simulink model "ISReferenceApplication"  (R2018a)
settings: Solver=FixedStepAuto  StartTime=0  StopTime=Tend  FixedStep=0.001  RelTol=5e-3
model workspace (MAT data in the model file):
  A_mu = 10
  B_reff = 8.386
  Cz = 7766.25
  DCT_Param : struct (value not decoded)
  D_reff = 0.25826
  Downshift_Speeds = [9.5625 12.9375 16.3125 19.6875 23.0625 26.4375 29.8125 33.1875 36.5625 39.9375 43.3125 46.6875 ... (28 elements, 4x7)]
  Pedal_Positions = [0.1 0.4 0.5 0.9]
  SUS : struct (value not decoded)
  Upshift_Speeds = [12.9375 16.3125 19.6875 33 26.4375 29.8125 33.1875 52.5 39.9375 43.3125 46.6875 77.25 ... (28 elements, 4x7)]
  VEH : struct (value not decoded)
  V_o = 16.7
  V_xlow = 1
  WH : struct (value not decoded)
  a = 1.4
  alpha_max = 1.5
  alpha_min = -1.5
  b = 1.8
  c_zo = 209651
  epsilon = 0.1
  h = 0.134
  path : struct (value not decoded)
  pio = 220000
  q_Fcx = 0
  q_Fz2 = 15.4
  q_Fzy = 0
  q_reo = 0.9974
  q_sx1 = -0.007764
  q_sx10 = 0.2824
  q_sx11 = 5.349
  q_sx12 = 0
  q_sx13 = 0
  q_sx14 = 0
  q_sx2 = 1.1915
  q_sx3 = 0.013948
  q_sx4 = 4.912
  q_sx5 = 1.02
  q_sx6 = 22.83
  q_sx7 = 0.7104
  q_sx8 = -0.023393
  q_sx9 = 0.6581
  q_sy1 = 0.00702
  q_sy2 = 0
  q_sy3 = 0.001515
  q_sy4 = 8.514e-05
  q_sy5 = 0
  q_sy6 = 0
  q_sy7 = 0.9008
  q_sy8 = -0.4089
  q_v1 = 0.0007742
  q_v2 = 0.04667
  r_Bx1 = 12.531
  r_Bx2 = 9.532
  r_Bx3 = 0
  r_By1 = 10.615
  r_By2 = 7.705
  r_By3 = 3.433e-06
  r_By4 = 0
  r_Cx1 = 1.019
  r_Cy1 = 1.0585
  r_Ex1 = -0.4487
  r_Ex2 = -0.4726
  r_Ey1 = 0.3132
  r_Ey2 = 7.63e-06
  r_Hx1 = 0.0002374
  r_Hy1 = 0.011646
  r_Hy2 = 7.63e-06
  r_Vy1 = 0.05654
  r_Vy2 = 7.63e-06
  r_Vy3 = 0
  r_Vy4 = 99.9
  r_Vy5 = 2
  r_Vy6 = 15.814
  r_o = 0.3135
  vehWidth = 2
  w = 1
undefined symbols (not defined in the file): Cok_1, Cok_2, Cok_3, Cok_4, Cok_5, Cok_6, Cok_7, Cok_8, Cok_9, Cout_1, Cout_2, Cout_3, Cout_4, Cout_5, Cout_6, Cout_7, Cout_8, Cout_9, Dout_1, Dout_2, Dout_3, Dout_4, Dout_5, Dout_6, Dout_7, Dout_8, Dout_9, F_1, F_2, F_3, F_4, F_5, F_6, F_7, F_8, F_9, Gd_1, Gd_2, Gd_3, Gd_4, Gd_5, Gd_6, Gd_7, Gd_8, Gd_9, Gok_1, Gok_2, Gok_3, Gok_4, Gok_5, Gok_6, Gok_7, Gok_8, Gok_9, Hd_1, Hd_2, Hd_3, Hd_4, Hd_5, Hd_6 ... (+64)
(part 3 of 3)

== system ISReferenceApplication/Subsystem_7/Subsystem/VH2P ==
  Velocities : Inport
  HeadingAngles : Inport  Port=2
  Iintial Velocities : Inport  Port=3
  Iintial HeadingAngles : Inport  Port=4
  Initial position : Inport  Port=5
  select_overlap : Inport  Port=6
  Delay1 : Delay  DelayLength=1  InitialConditionSource=Input port  InitialCondition=0  ExternalReset=Rising  SampleTime=Ts
      settings: InputPortMap=u0,r5,p4
  Delay2 : Delay  DelayLength=1  InitialConditionSource=Input port  InitialCondition=0  ExternalReset=Rising  SampleTime=Ts
      settings: InputPortMap=u0,r5,p4
  Delay3 : Delay  DelayLength=1  InitialConditionSource=Input port  InitialCondition=0  ExternalReset=Rising  SampleTime=Ts
      settings: InputPortMap=u0,r5,p4
  From Workspace : FromWorkspace  VariableName=T_sim  SampleTime=Ts
  Unit Delay3 : UnitDelay  SampleTime=Ts
  YV2P : MATLAB Function  TreatAsAtomicUnit=on  SystemSampleTime=Ts
  Position : Outport
  wires:
  Velocities/1 -> YV2P/1(Velocity), Delay1/1
  HeadingAngles/1 -> Delay3/1, YV2P/3(Yaw)
  Delay2/1 -> YV2P/7(Lastpostion)
  Initial position/1 -> Delay2/3
  Iintial Velocities/1 -> Delay1/3
  Iintial HeadingAngles/1 -> Delay3/3
  From Workspace/1 -> YV2P/5(Tsim), Unit Delay3/1
  Delay1/1 -> YV2P/2(LastVelocity)
  Delay3/1 -> YV2P/4(LastYaw)
  Unit Delay3/1 -> YV2P/6(LastTsim)
  YV2P/1(Position) -> Delay2/1, Position/1
  select_overlap/1 -> Delay2/2, Delay1/2, Delay3/2

== system ISReferenceApplication/Subsystem_7/Subsystem/YV_update ==
  XY_sim : Inport
  Velocity_sim : Inport  Port=2
  Heading_sim : Inport  Port=3
  Constant : Constant  Value=Ts  SampleTime=Ts
  From Workspace1 : FromWorkspace  VariableName=T_sim  SampleTime=Ts
  From Workspace3 : FromWorkspace  VariableName=XY_Ref_Upd  SampleTime=Ts
  YV_update : MATLAB Function  TreatAsAtomicUnit=on  SystemSampleTime=Ts
  Velocity_updated : Outport
  Heading_updated : Outport  Port=2
  wires:
  YV_update/1(Velocity_updated) -> Velocity_updated/1
  From Workspace3/1 -> YV_update/1(XYplot_ref)
  YV_update/2(Heading_updated) -> Heading_updated/1
  From Workspace1/1 -> YV_update/6(Tsim)
  XY_sim/1 -> YV_update/2(XYplot_sim)
  Velocity_sim/1 -> YV_update/3(Velocity_sim)
  Heading_sim/1 -> YV_update/4(Heading_sim)
  Constant/1 -> YV_update/5(Ts)

== system ISReferenceApplication/Subsystem_8/Subsystem/MPC_of_simulator_8 ==
  Velocity_updated : Inport  SampleTime=Ts  LockScale=on
  Heading_updated : Inport  Port=2  SampleTime=Ts  LockScale=on
  select_MPC : Inport  Port=3  SampleTime=Ts  LockScale=on
  select_overlap : Inport  Port=4  SampleTime=Ts  LockScale=on
  U(k-1) : Inport  Port=5  SampleTime=Ts  LockScale=on
  Xhat : Inport  Port=6
  Clock : Clock
  Constant1 : Constant  Value=M  VectorParams1D=off  SampleTime=-1
  Constant2 : Constant  Value=Np  SampleTime=-1
  Constant3 : Constant  Value=JE_8  VectorParams1D=off  SampleTime=-1
  Constant4 : Constant  Value=Qc_8  VectorParams1D=off  SampleTime=-1
  Constant5 : Constant  Value=phi_8  VectorParams1D=off  SampleTime=-1
  Constant6 : Constant  Value=Tend  SampleTime=-1
  F_Middle : Gain  Gain=F_8  Multiplication=Matrix(K*u) (u vector)
  From Workspace6 : FromWorkspace  VariableName=Rs  SampleTime=Ts
  HQP : MATLAB Function  TreatAsAtomicUnit=on  SystemSampleTime=Ts
  Resettable Delay2 : Delay  DelayLength=1  InitialConditionSource=Input port  ExternalReset=Rising  SampleTime=Ts
      settings: InputPortMap=u0,r5,p4
  r(k+1) : Outport
  U : Outport  Port=2
  wires:
  HQP/2(U) -> Resettable Delay2/1, U/1
  Xhat/1 -> F_Middle/1
  Constant4/1 -> HQP/4(Qc)
  Constant5/1 -> HQP/2(phi)
  Constant3/1 -> HQP/1(JE)
  Constant2/1 -> HQP/6(Np)
  Constant1/1 -> HQP/5(M)
  Clock/1 -> HQP/10(Tsim)
  F_Middle/1 -> HQP/3(Fxh)
  From Workspace6/1 -> HQP/9(Rs)
  Heading_updated/1 -> HQP/7(Heading_updated)
  Velocity_updated/1 -> HQP/8(Velocity_updated)
  HQP/1(r) -> r(k+1)/1
  select_MPC/1 -> HQP/11(select_MPC)
  Resettable Delay2/1 -> HQP/13(U_delay)
  select_overlap/1 -> Resettable Delay2/2
  U(k-1)/1 -> Resettable Delay2/3
  Constant6/1 -> HQP/12(Tend)

== system ISReferenceApplication/Subsystem_8/Subsystem/VH2P ==
  Velocities : Inport
  HeadingAngles : Inport  Port=2
  Iintial Velocities : Inport  Port=3
  Iintial HeadingAngles : Inport  Port=4
  Initial position : Inport  Port=5
  select_overlap : Inport  Port=6
  Delay1 : Delay  DelayLength=1  InitialConditionSource=Input port  InitialCondition=0  ExternalReset=Rising  SampleTime=Ts
      settings: InputPortMap=u0,r5,p4
  Delay2 : Delay  DelayLength=1  InitialConditionSource=Input port  InitialCondition=0  ExternalReset=Rising  SampleTime=Ts
      settings: InputPortMap=u0,r5,p4
  Delay3 : Delay  DelayLength=1  InitialConditionSource=Input port  InitialCondition=0  ExternalReset=Rising  SampleTime=Ts
      settings: InputPortMap=u0,r5,p4
  From Workspace : FromWorkspace  VariableName=T_sim  SampleTime=Ts
  Unit Delay3 : UnitDelay  SampleTime=Ts
  YV2P : MATLAB Function  TreatAsAtomicUnit=on  SystemSampleTime=Ts
  Position : Outport
  wires:
  Velocities/1 -> YV2P/1(Velocity), Delay1/1
  HeadingAngles/1 -> Delay3/1, YV2P/3(Yaw)
  Delay2/1 -> YV2P/7(Lastpostion)
  Initial position/1 -> Delay2/3
  Iintial Velocities/1 -> Delay1/3
  Iintial HeadingAngles/1 -> Delay3/3
  From Workspace/1 -> YV2P/5(Tsim), Unit Delay3/1
  Delay1/1 -> YV2P/2(LastVelocity)
  Delay3/1 -> YV2P/4(LastYaw)
  Unit Delay3/1 -> YV2P/6(LastTsim)
  YV2P/1(Position) -> Delay2/1, Position/1
  select_overlap/1 -> Delay2/2, Delay1/2, Delay3/2

== system ISReferenceApplication/Subsystem_8/Subsystem/YV_update ==
  XY_sim : Inport
  Velocity_sim : Inport  Port=2
  Heading_sim : Inport  Port=3
  Constant : Constant  Value=Ts  SampleTime=Ts
  From Workspace1 : FromWorkspace  VariableName=T_sim  SampleTime=Ts
  From Workspace3 : FromWorkspace  VariableName=XY_Ref_Upd  SampleTime=Ts
  YV_update : MATLAB Function  TreatAsAtomicUnit=on  SystemSampleTime=Ts
  Velocity_updated : Outport
  Heading_updated : Outport  Port=2
  wires:
  YV_update/1(Velocity_updated) -> Velocity_updated/1
  From Workspace3/1 -> YV_update/1(XYplot_ref)
  YV_update/2(Heading_updated) -> Heading_updated/1
  From Workspace1/1 -> YV_update/6(Tsim)
  XY_sim/1 -> YV_update/2(XYplot_sim)
  Velocity_sim/1 -> YV_update/3(Velocity_sim)
  Heading_sim/1 -> YV_update/4(Heading_sim)
  Constant/1 -> YV_update/5(Ts)

== system ISReferenceApplication/Subsystem_9/Subsystem/MPC_of_simulator_9 ==
  Velocity_updated : Inport  SampleTime=Ts  LockScale=on
  Heading_updated : Inport  Port=2  SampleTime=Ts  LockScale=on
  select_MPC : Inport  Port=3  SampleTime=Ts  LockScale=on
  select_overlap : Inport  Port=4  SampleTime=Ts  LockScale=on
  U(k-1) : Inport  Port=5  SampleTime=Ts  LockScale=on
  Xhat : Inport  Port=6
  Clock : Clock
  Constant1 : Constant  Value=M  VectorParams1D=off  SampleTime=-1
  Constant2 : Constant  Value=Np  SampleTime=-1
  Constant3 : Constant  Value=JE_9  VectorParams1D=off  SampleTime=-1
  Constant4 : Constant  Value=Qc_9  VectorParams1D=off  SampleTime=-1
  Constant5 : Constant  Value=phi_9  VectorParams1D=off  SampleTime=-1
  Constant6 : Constant  Value=Tend  SampleTime=-1
  F_Middle : Gain  Gain=F_9  Multiplication=Matrix(K*u) (u vector)
  From Workspace6 : FromWorkspace  VariableName=Rs  SampleTime=Ts
  HQP : MATLAB Function  TreatAsAtomicUnit=on  SystemSampleTime=Ts
  Resettable Delay2 : Delay  DelayLength=1  InitialConditionSource=Input port  ExternalReset=Rising  SampleTime=Ts
      settings: InputPortMap=u0,r5,p4
  r(k+1) : Outport
  U : Outport  Port=2
  wires:
  HQP/2(U) -> Resettable Delay2/1, U/1
  Xhat/1 -> F_Middle/1
  Constant4/1 -> HQP/4(Qc)
  Constant5/1 -> HQP/2(phi)
  Constant3/1 -> HQP/1(JE)
  Constant2/1 -> HQP/6(Np)
  Constant1/1 -> HQP/5(M)
  Clock/1 -> HQP/10(Tsim)
  F_Middle/1 -> HQP/3(Fxh)
  From Workspace6/1 -> HQP/9(Rs)
  Heading_updated/1 -> HQP/7(Heading_updated)
  Velocity_updated/1 -> HQP/8(Velocity_updated)
  HQP/1(r) -> r(k+1)/1
  select_MPC/1 -> HQP/11(select_MPC)
  Resettable Delay2/1 -> HQP/13(U_delay)
  select_overlap/1 -> Resettable Delay2/2
  U(k-1)/1 -> Resettable Delay2/3
  Constant6/1 -> HQP/12(Tend)

== system ISReferenceApplication/Subsystem_9/Subsystem/VH2P ==
  Velocities : Inport
  HeadingAngles : Inport  Port=2
  Iintial Velocities : Inport  Port=3
  Iintial HeadingAngles : Inport  Port=4
  Initial position : Inport  Port=5
  select_overlap : Inport  Port=6
  Delay1 : Delay  DelayLength=1  InitialConditionSource=Input port  InitialCondition=0  ExternalReset=Rising  SampleTime=Ts
      settings: InputPortMap=u0,r5,p4
  Delay2 : Delay  DelayLength=1  InitialConditionSource=Input port  InitialCondition=0  ExternalReset=Rising  SampleTime=Ts
      settings: InputPortMap=u0,r5,p4
  Delay3 : Delay  DelayLength=1  InitialConditionSource=Input port  InitialCondition=0  ExternalReset=Rising  SampleTime=Ts
      settings: InputPortMap=u0,r5,p4
  From Workspace : FromWorkspace  VariableName=T_sim  SampleTime=Ts
  Unit Delay3 : UnitDelay  SampleTime=Ts
  YV2P : MATLAB Function  TreatAsAtomicUnit=on  SystemSampleTime=Ts
  Position : Outport
  wires:
  Velocities/1 -> YV2P/1(Velocity), Delay1/1
  HeadingAngles/1 -> Delay3/1, YV2P/3(Yaw)
  Delay2/1 -> YV2P/7(Lastpostion)
  Initial position/1 -> Delay2/3
  Iintial Velocities/1 -> Delay1/3
  Iintial HeadingAngles/1 -> Delay3/3
  From Workspace/1 -> YV2P/5(Tsim), Unit Delay3/1
  Delay1/1 -> YV2P/2(LastVelocity)
  Delay3/1 -> YV2P/4(LastYaw)
  Unit Delay3/1 -> YV2P/6(LastTsim)
  YV2P/1(Position) -> Delay2/1, Position/1
  select_overlap/1 -> Delay2/2, Delay1/2, Delay3/2

== system ISReferenceApplication/Subsystem_9/Subsystem/YV_update ==
  XY_sim : Inport
  Velocity_sim : Inport  Port=2
  Heading_sim : Inport  Port=3
  Constant : Constant  Value=Ts  SampleTime=Ts
  From Workspace1 : FromWorkspace  VariableName=T_sim  SampleTime=Ts
  From Workspace3 : FromWorkspace  VariableName=XY_Ref_Upd  SampleTime=Ts
  YV_update : MATLAB Function  TreatAsAtomicUnit=on  SystemSampleTime=Ts
  Velocity_updated : Outport
  Heading_updated : Outport  Port=2
  wires:
  YV_update/1(Velocity_updated) -> Velocity_updated/1
  From Workspace3/1 -> YV_update/1(XYplot_ref)
  YV_update/2(Heading_updated) -> Heading_updated/1
  From Workspace1/1 -> YV_update/6(Tsim)
  XY_sim/1 -> YV_update/2(XYplot_sim)
  Velocity_sim/1 -> YV_update/3(Velocity_sim)
  Heading_sim/1 -> YV_update/4(Heading_sim)
  Constant/1 -> YV_update/5(Ts)

== matlab function ISReferenceApplication/Subsystem_6/Subsystem/MPC_of_simulator_6/HQP ==
  data: r output; JE input; phi input; Fxh input; Qc input; U output; M input; Np input; Heading_updated input; Velocity_updated input; Rs input; Tsim input; select_MPC input; Tend input; U_delay input; select_overlap input
function [r,U] = HQP(JE ,phi,Fxh ,Qc ,M ,Np,Heading_updated ,Velocity_updated ,Rs ,Tsim, select_MPC, Tend, U_delay, select_overlap)
u1_max = 3*pi; u1_min = -3*pi;
u2_max =  1; u2_min = -1;
du1_inc = 3*pi;du1_dec = 3*pi;
du2_inc =  1;du2_dec =  1;
U_max = []; U_min = [];
for i = 1:Np
    U_max = [U_max; [u1_max; u2_max]];
    U_min = [U_min; [-u1_min; -u2_min]];
end

dU_plus = []; dU_minus = [];
for i = 1:Np
    dU_plus = [dU_plus; [U_delay(1) + du1_inc; U_delay(2) + du2_inc]];
    dU_minus = [dU_minus; [-U_delay(1) + du1_dec; -U_delay(2) + du2_dec;]];
end
N = [U_max;
      U_min;
      dU_plus;
      dU_minus;          
     ];
if Tsim > 0 %&& select_MPC~=1 %&& select_overlap~=1 
    for i = 1: Np
        Rs(2*i,:) = Heading_updated(i,:);
        Rs(2*i-1,:) = Velocity_updated(i,:);
    end
end
JF = -2*phi'*Qc*(Rs-Fxh);
[u,lambda]= HQP(JE,JF,M,N);
U = u(1:2);
r = Rs(1:2,:);
end

== matlab function ISReferenceApplication/Subsystem_6/Subsystem/VH2P/YV2P ==
  data: Velocity input; LastVelocity input; Yaw input; LastYaw input; Tsim input; LastTsim input; Lastpostion input; Position output
function Position  = YV2P(Velocity, LastVelocity, Yaw, LastYaw, Tsim, LastTsim, Lastpostion)
if Tsim >= 0.1
    Position = zeros(2,1);
    X0 = Lastpostion(1,:); Y0 = Lastpostion(2,:);
    Vx = [LastVelocity*cos(LastYaw); Velocity*cos(Yaw)];
    Vy = [LastVelocity*sin(LastYaw); Velocity*sin(Yaw)];
    Yaw_sim = [LastYaw; Yaw];
    T_sample =[LastTsim; Tsim];
    [ X_tmp, Y_tmp] = YV2P( T_sample, X0, Y0, Vx, Vy, Yaw_sim, zeros(2,1) );
    Position = [X_tmp(end,:); Y_tmp(end,:)];
else
    Position = [0; 0];
end

end

== matlab function ISReferenceApplication/Subsystem_6/Subsystem/YV_update/YV_update ==
  data: XYplot_ref input; Velocity_updated output; XYplot_sim input; Velocity_sim input; Heading_sim input; Ts input; Tsim input; Heading_updated output
function [Velocity_updated, Heading_updated] = VY_update(XYplot_ref, XYplot_sim, Velocity_sim, Heading_sim, Ts, Tsim)
Np = 6;
 disp(sprintf('Simulation time : %2.1f sec',Tsim)) 
 Heading_updated = zeros(Np,1); Velocity_updated = zeros(Np,1);
coder.extrinsic('P2YV');
T = []; 
for j = 1:Np+1
    T = [T; Tsim+(j-1)*Ts];
end
X = [];
for i = 1:Np
    X = [X; XYplot_ref(2*i-1,:)];
end
Y = [];
for i = 1:Np
    Y = [Y; XYplot_ref(2*i,:)];
end

X = [XYplot_sim(1,:); X];
Y = [XYplot_sim(2,:); Y];   
Vx0 = Velocity_sim*cos(Heading_sim);
Vy0 = Velocity_sim*sin(Heading_sim);
Yaw0 = Heading_sim;

[Velocity_updated, Heading_updated] = P2YV(0,0, T , X , Y , Vx0 , Vy0 , Yaw0, Np, 0, 0 );
end

== matlab function ISReferenceApplication/Subsystem_3/Subsystem/MPC_of_simulator_3/HQP ==
  data: r output; JE input; phi input; Fxh input; Qc input; U output; M input; Np input; Heading_updated input; Velocity_updated input; Rs input; Tsim input; select_MPC input; Tend input; U_delay input; select_overlap input
function [r,U] = HQP(JE ,phi,Fxh ,Qc ,M ,Np,Heading_updated ,Velocity_updated ,Rs ,Tsim, select_MPC, Tend, U_delay, select_overlap)
u1_max = 3*pi; u1_min = -3*pi;
u2_max =  1; u2_min = -1;
du1_inc = 3*pi;du1_dec = 3*pi;
du2_inc =  1;du2_dec =  1;
U_max = []; U_min = [];
for i = 1:Np
    U_max = [U_max; [u1_max; u2_max]];
    U_min = [U_min; [-u1_min; -u2_min]];
end

dU_plus = []; dU_minus = [];
for i = 1:Np
    dU_plus = [dU_plus; [U_delay(1) + du1_inc; U_delay(2) + du2_inc]];
    dU_minus = [dU_minus; [-U_delay(1) + du1_dec; -U_delay(2) + du2_dec;]];
end
N = [U_max;
      U_min;
      dU_plus;
      dU_minus;          
     ];
if Tsim > 0 %&& select_overlap~=1 && select_MPC~=1
    for i = 1: Np
        Rs(2*i,:) = Heading_updated(i,:);
        Rs(2*i-1,:) = Velocity_updated(i,:);
    end
end
JF = -2*phi'*Qc*(Rs-Fxh);
[u,lambda]= HQP(JE,JF,M,N);

U = u(1:2);
r = Rs(1:2,:);
end

== matlab function ISReferenceApplication/Subsystem_3/Subsystem/VH2P/YV2P ==
  data: Velocity input; LastVelocity input; Yaw input; LastYaw input; Tsim input; LastTsim input; Lastpostion input; Position output
function Position  = YV2P(Velocity, LastVelocity, Yaw, LastYaw, Tsim, LastTsim, Lastpostion)
if Tsim >= 0.1
    Position = zeros(2,1);
    X0 = Lastpostion(1,:); Y0 = Lastpostion(2,:);
    Vx = [LastVelocity*cos(LastYaw); Velocity*cos(Yaw)];
    Vy = [LastVelocity*sin(LastYaw); Velocity*sin(Yaw)];
    Yaw_sim = [LastYaw; Yaw];
    T_sample =[LastTsim; Tsim];
    [ X_tmp, Y_tmp] = YV2P( T_sample, X0, Y0, Vx, Vy, Yaw_sim, zeros(2,1) );
    Position = [X_tmp(end,:); Y_tmp(end,:)];
else
    Position = [0; 0];
end

end

== matlab function ISReferenceApplication/Subsystem_4/Subsystem/MPC_of_simulator_4/HQP ==
  data: r output; JE input; phi input; Fxh input; Qc input; U output; M input; Np input; Heading_updated input; Velocity_updated input; Rs input; Tsim input; select_MPC input; Tend input; U_delay input; select_overlap input
function [r,U] = HQP(JE ,phi,Fxh ,Qc ,M ,Np,Heading_updated ,Velocity_updated ,Rs ,Tsim, select_MPC, Tend, U_delay, select_overlap)
u1_max = 3*pi; u1_min = -3*pi;
u2_max =  1; u2_min = -1;
du1_inc = 3*pi;du1_dec = 3*pi;
du2_inc =  1;du2_dec =  1;
U_max = []; U_min = [];
for i = 1:Np
    U_max = [U_max; [u1_max; u2_max]];
    U_min = [U_min; [-u1_min; -u2_min]];
end

dU_plus = []; dU_minus = [];
for i = 1:Np
    dU_plus = [dU_plus; [U_delay(1) + du1_inc; U_delay(2) + du2_inc]];
    dU_minus = [dU_minus; [-U_delay(1) + du1_dec; -U_delay(2) + du2_dec;]];
end
N = [U_max;
      U_min;
      dU_plus;
      dU_minus;          
     ];
 
if Tsim > 0 && select_MPC~=1 %&& select_overlap~=1
    for i = 1: Np
        Rs(2*i,:) = Heading_updated(i,:);
        Rs(2*i-1,:) = Velocity_updated(i,:);
    end
end

JF = -2*phi'*Qc*(Rs-Fxh);
[u,lambda]= HQP(JE,JF,M,N);
U = u(1:2);
r = Rs(1:2,:);
end

== matlab function ISReferenceApplication/Subsystem_5/Subsystem/MPC_of_simulator_5/HQP ==
  data: r output; JE input; phi input; Fxh input; Qc input; U output; M input; Np input; Heading_updated input; Velocity_updated input; Rs input; Tsim input; select_MPC input; Tend input; U_delay input; select_overlap input
function [r,U] = HQP(JE ,phi,Fxh ,Qc ,M ,Np,Heading_updated ,Velocity_updated ,Rs ,Tsim, select_MPC, Tend, U_delay, select_overlap)
u1_max = 3*pi; u1_min = -3*pi;
u2_max =  1; u2_min = -1;
du1_inc = 3*pi;du1_dec = 3*pi;
du2_inc =  1;du2_dec =  1;
U_max = []; U_min = [];
for i = 1:Np
    U_max = [U_max; [u1_max; u2_max]];
    U_min = [U_min; [-u1_min; -u2_min]];
end

dU_plus = []; dU_minus = [];
for i = 1:Np
    dU_plus = [dU_plus; [U_delay(1) + du1_inc; U_delay(2) + du2_inc]];
    dU_minus = [dU_minus; [-U_delay(1) + du1_dec; -U_delay(2) + du2_dec;]];
end
N = [U_max;
      U_min;
      dU_plus;
      dU_minus;          
     ];
if Tsim > 0 %&& select_overlap~=1 && select_MPC~=1
    for i = 1: Np
        Rs(2*i,:) = Heading_updated(i,:);
        Rs(2*i-1,:) = Velocity_updated(i,:);
    end
end
JF = -2*phi'*Qc*(Rs-Fxh);
[u,lambda]= HQP(JE,JF,M,N);
U = u(1:2);
r = Rs(1:2,:);
end

== matlab function ISReferenceApplication/Subsystem_7/Subsystem/MPC_of_simulator_7/HQP ==
  data: r output; JE input; phi input; Fxh input; Qc input; U output; M input; Np input; Heading_updated input; Velocity_updated input; Rs input; Tsim input; select_MPC input; Tend input; U_delay input; select_overlap input
function [r,U] = HQP(JE ,phi,Fxh ,Qc ,M ,Np,Heading_updated ,Velocity_updated ,Rs ,Tsim, select_MPC, Tend, U_delay, select_overlap)
u1_max = 3*pi; u1_min = -3*pi;
u2_max =  1; u2_min = -1;
du1_inc = 3*pi;du1_dec = 3*pi;
du2_inc =  1;du2_dec =  1;
U_max = []; U_min = [];
for i = 1:Np
    U_max = [U_max; [u1_max; u2_max]];
    U_min = [U_min; [-u1_min; -u2_min]];
end

dU_plus = []; dU_minus = [];
for i = 1:Np
    dU_plus = [dU_plus; [U_delay(1) + du1_inc; U_delay(2) + du2_inc]];
    dU_minus = [dU_minus; [-U_delay(1) + du1_dec; -U_delay(2) + du2_dec;]];
end
N = [U_max;
      U_min;
      dU_plus;
      dU_minus;          
     ];
if Tsim > 0 %&& select_overlap~=1 && select_MPC~=1
    for i = 1: Np
        Rs(2*i,:) = Heading_updated(i,:);
        Rs(2*i-1,:) = Velocity_updated(i,:);
    end
end
JF = -2*phi'*Qc*(Rs-Fxh);
[u,lambda]= HQP(JE,JF,M,N);
U = u(1:2);
r = Rs(1:2,:);
end

== matlab function ISReferenceApplication/Subsystem_8/Subsystem/MPC_of_simulator_8/HQP ==
  data: r output; JE input; phi input; Fxh input; Qc input; U output; M input; Np input; Heading_updated input; Velocity_updated input; Rs input; Tsim input; select_MPC input; Tend input; U_delay input; select_overlap input
function [r,U] = HQP(JE ,phi,Fxh ,Qc ,M ,Np,Heading_updated ,Velocity_updated ,Rs ,Tsim, select_MPC, Tend, U_delay, select_overlap)
u1_max = 3*pi; u1_min = -3*pi;
u2_max =  1; u2_min = -1;
du1_inc = 3*pi;du1_dec = 3*pi;
du2_inc =  1;du2_dec =  1;
U_max = []; U_min = [];
for i = 1:Np
    U_max = [U_max; [u1_max; u2_max]];
    U_min = [U_min; [-u1_min; -u2_min]];
end

dU_plus = []; dU_minus = [];
for i = 1:Np
    dU_plus = [dU_plus; [U_delay(1) + du1_inc; U_delay(2) + du2_inc]];
    dU_minus = [dU_minus; [-U_delay(1) + du1_dec; -U_delay(2) + du2_dec;]];
end
N = [U_max;
      U_min;
      dU_plus;
      dU_minus;          
     ];
if Tsim > 0 %&& select_overlap~=1 && select_MPC~=1
    for i = 1: Np
        Rs(2*i,:) = Heading_updated(i,:);
        Rs(2*i-1,:) = Velocity_updated(i,:);
    end
end
JF = -2*phi'*Qc*(Rs-Fxh);
[u,lambda]= HQP(JE,JF,M,N);
U = u(1:2);
r = Rs(1:2,:);
end

== matlab function ISReferenceApplication/Subsystem_9/Subsystem/MPC_of_simulator_9/HQP ==
  data: r output; JE input; phi input; Fxh input; Qc input; U output; M input; Np input; Heading_updated input; Velocity_updated input; Rs input; Tsim input; select_MPC input; Tend input; U_delay input
function [r,U] = HQP(JE ,phi,Fxh ,Qc ,M ,Np,Heading_updated ,Velocity_updated ,Rs ,Tsim, select_MPC, Tend, U_delay)
u1_max = 3*pi; u1_min = -3*pi;
u2_max =  1; u2_min = -1;
du1_inc = 3*pi;du1_dec = 3*pi;
du2_inc =  1;du2_dec =  1;
U_max = []; U_min = [];
for i = 1:Np
    U_max = [U_max; [u1_max; u2_max]];
    U_min = [U_min; [-u1_min; -u2_min]];
end

dU_plus = []; dU_minus = [];
for i = 1:Np
    dU_plus = [dU_plus; [U_delay(1) + du1_inc; U_delay(2) + du2_inc]];
    dU_minus = [dU_minus; [-U_delay(1) + du1_dec; -U_delay(2) + du2_dec;]];
end
N = [U_max;
      U_min;
      dU_plus;
      dU_minus;          
     ];
if Tsim > 0
    for i = 1: Np
        Rs(2*i,:) = Heading_updated(i,:);
        Rs(2*i-1,:) = Velocity_updated(i,:);
    end
end
JF = -2*phi'*Qc*(Rs-Fxh);
[u,lambda]= HQP(JE,JF,M,N);
U = u(1:2);
r = Rs(1:2,:);
end

== matlab function ISReferenceApplication/Mpc_block1/Mpc ==
  data: U_delay input; select_MPC input; JE input; JF_part input; Fxh input; M input; Np input; U_min input; U_max input; Heading_updated input; Velocity_updated input; Rs input; Tsim input; U output; r output; lambda output; Tend input; Ts input
function [U, r, lambda] = ABC(U_delay, select_MPC, JE, JF_part, Fxh, M, Np, U_min, U_max, Heading_updated, Velocity_updated, Rs, Tsim, Tend, Ts)
U = zeros(2,1);
du1_inc = 3*pi;du1_dec = 3*pi;
du2_inc = 1;du2_dec = 1;
dU_plus = []; dU_minus = [];
for i = 1:Np
    dU_plus = [dU_plus; [U_delay(1) + du1_inc; U_delay(2) + du2_inc]];
    dU_minus = [dU_minus; [-U_delay(1) + du1_dec; -U_delay(2) + du2_dec;]];
end

N = [U_max;
      U_min;
      dU_plus;
      dU_minus;          
     ];
 
if Tsim > 0 && select_MPC ~= 4 %&& select_MPC ~= 5 %&& select_MPC ~= 6 %&& select_MPC~=8
    for i = 1: Np  
        Rs(2*i-1,:) = Velocity_updated(i,:);
        Rs(2*i,:) = Heading_updated(i,:);
    end
end

JF = JF_part*(Rs-Fxh);
[u,lambda]= HQP(JE,JF,M,N);
U = u(1:2);
r = Rs(1:2,:);
end

== matlab function ISReferenceApplication/Subsystem_1/Subsystem/MPC_of_simulator_1/HQP ==
  data: r output; JE input; phi input; Fxh input; Qc input; U output; M input; Np input; Heading_updated input; Velocity_updated input; Rs input; Tsim input; select_MPC input; Tend input; U_delay input; select_overlap input
function [r,U] = HQP(JE ,phi,Fxh ,Qc ,M ,Np,Heading_updated ,Velocity_updated ,Rs ,Tsim, select_MPC, Tend, U_delay, select_overlap)
u1_max = 3*pi; u1_min = -3*pi;
u2_max =  1; u2_min = -1;
du1_inc = 3*pi;du1_dec = 3*pi;
du2_inc =  1;du2_dec =  1;
U_max = []; U_min = [];
for i = 1:Np
    U_max = [U_max; [u1_max; u2_max]];
    U_min = [U_min; [-u1_min; -u2_min]];
end

dU_plus = []; dU_minus = [];
for i = 1:Np
    dU_plus = [dU_plus; [U_delay(1) + du1_inc; U_delay(2) + du2_inc]];
    dU_minus = [dU_minus; [-U_delay(1) + du1_dec; -U_delay(2) + du2_dec;]];
end
N = [U_max;
      U_min;
      dU_plus;
      dU_minus;          
     ];
if Tsim > 0 %&& select_overlap~=1 && select_MPC~=1
    for i = 1: Np
        Rs(2*i,:) = Heading_updated(i,:);
        Rs(2*i-1,:) = Velocity_updated(i,:);
    end
end
JF = -2*phi'*Qc*(Rs-Fxh);
[u,lambda]= HQP(JE,JF,M,N);
U = u(1:2);
r = Rs(1:2,:);
end

== matlab function ISReferenceApplication/Subsystem_1/Subsystem/VH2P/YV2P ==
  data: Velocity input; LastVelocity input; Yaw input; LastYaw input; Tsim input; LastTsim input; Lastpostion input; Position output
function Position  = YV2P(Velocity, LastVelocity, Yaw, LastYaw, Tsim, LastTsim, Lastpostion)
if Tsim >= 0.1
    Position = zeros(2,1);
    X0 = Lastpostion(1,:); Y0 = Lastpostion(2,:);
    Vx = [LastVelocity*cos(LastYaw); Velocity*cos(Yaw)];
    Vy = [LastVelocity*sin(LastYaw); Velocity*sin(Yaw)];
    Yaw_sim = [LastYaw; Yaw];
    T_sample =[LastTsim; Tsim];
    [ X_tmp, Y_tmp] = YV2P( T_sample, X0, Y0, Vx, Vy, Yaw_sim, zeros(2,1) );
    Position = [X_tmp(end,:); Y_tmp(end,:)];
else
    Position = [0; 0];
end

end

== matlab function ISReferenceApplication/Subsystem_1/Subsystem/YV_update/YV_update ==
  data: XYplot_ref input; Velocity_updated output; XYplot_sim input; Velocity_sim input; Heading_sim input; Ts input; Tsim input; Heading_updated output
function [Velocity_updated, Heading_updated] = VY_update(XYplot_ref, XYplot_sim, Velocity_sim, Heading_sim, Ts, Tsim)
Np = 6;
 disp(sprintf('Simulation time : %2.1f sec',Tsim)) 
 Heading_updated = zeros(Np,1); Velocity_updated = zeros(Np,1);
coder.extrinsic('P2YV');
T = []; 
for j = 1:Np+1
    T = [T; Tsim+(j-1)*Ts];
end
X = [];
for i = 1:Np
    X = [X; XYplot_ref(2*i-1,:)];
end
Y = [];
for i = 1:Np
    Y = [Y; XYplot_ref(2*i,:)];
end

X = [XYplot_sim(1,:); X];
Y = [XYplot_sim(2,:); Y];   
Vx0 = Velocity_sim*cos(Heading_sim);
Vy0 = Velocity_sim*sin(Heading_sim);
Yaw0 = Heading_sim;

[Velocity_updated, Heading_updated] = P2YV(0,0, T , X , Y , Vx0 , Vy0 , Yaw0, Np, 0, 0 );
end

== matlab function ISReferenceApplication/Subsystem_2/Subsystem/MPC_of_simulator_2/HQP ==
  data: r output; JE input; phi input; Fxh input; Qc input; U output; M input; Np input; Heading_updated input; Velocity_updated input; Rs input; Tsim input; select_MPC input; Tend input; U_delay input
function [r,U] = HQP(JE ,phi,Fxh ,Qc ,M ,Np,Heading_updated ,Velocity_updated ,Rs ,Tsim, select_MPC, Tend, U_delay)
u1_max = 3*pi; u1_min = -3*pi;
u2_max =  1; u2_min = -1;
du1_inc = 3*pi;du1_dec = 3*pi;
du2_inc =  1;du2_dec =  1;
U_max = []; U_min = [];
for i = 1:Np
    U_max = [U_max; [u1_max; u2_max]];
    U_min = [U_min; [-u1_min; -u2_min]];
end

dU_plus = []; dU_minus = [];
for i = 1:Np
    dU_plus = [dU_plus; [U_delay(1) + du1_inc; U_delay(2) + du2_inc]];
    dU_minus = [dU_minus; [-U_delay(1) + du1_dec; -U_delay(2) + du2_dec;]];
end
N = [U_max;
      U_min;
      dU_plus;
      dU_minus;          
     ];
if Tsim > 0
    for i = 1: Np
        Rs(2*i,:) = Heading_updated(i,:);
        Rs(2*i-1,:) = Velocity_updated(i,:);
    end
end
JF = -2*phi'*Qc*(Rs-Fxh);
[u,lambda]= HQP(JE,JF,M,N);
U = u(1:2);
r = Rs(1:2,:);
end

== matlab function ISReferenceApplication/YV_update_Np1/MATLAB Function2 ==
  data: XY_ref input; Velocity_updated output; XYplot_sim input; Velocity_sim input; Yaw_sim input; Tsim input; Heading_updated output
function [Velocity_updated, Heading_updated] = VY_update(XY_ref, XYplot_sim, Velocity_sim, Yaw_sim, Tsim)
disp(sprintf('Simulation time : %2.1f sec',Tsim)) 
Ts = 0.1;
Np = 6;
Heading_updated = zeros(Np,1); Velocity_updated = zeros(Np,1);
coder.extrinsic('P2YV');

T_sample = []; 
for j = 1:Np+1
    T_sample = [T_sample; Tsim+(j-1)*Ts];
end
X = [];
for i = 1:Np
    X = [X; XY_ref(2*i-1,:)];
end
Y = [];
for i = 1:Np
    Y = [Y; XY_ref(2*i,:)];
end

X = [XYplot_sim(1,:); X];
Y = [XYplot_sim(2,:); Y];
Vx0 = Velocity_sim*cos(Yaw_sim);
Vy0 = Velocity_sim*sin(Yaw_sim);
Yaw0 = Yaw_sim;

[Velocity_updated, Heading_updated] = P2YV(0,0, T_sample , X , Y , Vx0 , Vy0 , Yaw0, Np, 0, 0 );

end

== matlab function ISReferenceApplication/Subsystem_2/Subsystem/VH2P/YV2P ==
  data: Velocity input; LastVelocity input; Yaw input; LastYaw input; Tsim input; LastTsim input; Lastpostion input; Position output
function Position  = YV2P(Velocity, LastVelocity, Yaw, LastYaw, Tsim, LastTsim, Lastpostion)
if Tsim >= 0.1
    Position = zeros(2,1);
    X0 = Lastpostion(1,:); Y0 = Lastpostion(2,:);
    Vx = [LastVelocity*cos(LastYaw); Velocity*cos(Yaw)];
    Vy = [LastVelocity*sin(LastYaw); Velocity*sin(Yaw)];
    Yaw_sim = [LastYaw; Yaw];
    T_sample =[LastTsim; Tsim];
    [ X_tmp, Y_tmp] = YV2P( T_sample, X0, Y0, Vx, Vy, Yaw_sim, zeros(2,1) );
    Position = [X_tmp(end,:); Y_tmp(end,:)];
else
    Position = [0; 0];
end

end

== matlab function ISReferenceApplication/Subsystem_2/Subsystem/YV_update/YV_update ==
  data: XYplot_ref input; Velocity_updated output; XYplot_sim input; Velocity_sim input; Heading_sim input; Ts input; Tsim input; Heading_updated output
function [Velocity_updated, Heading_updated] = VY_update(XYplot_ref, XYplot_sim, Velocity_sim, Heading_sim, Ts, Tsim)
Np = 6;
 disp(sprintf('Simulation time : %2.1f sec',Tsim)) 
 Heading_updated = zeros(Np,1); Velocity_updated = zeros(Np,1);
coder.extrinsic('P2YV');
T = []; 
for j = 1:Np+1
    T = [T; Tsim+(j-1)*Ts];
end
X = [];
for i = 1:Np
    X = [X; XYplot_ref(2*i-1,:)];
end
Y = [];
for i = 1:Np
    Y = [Y; XYplot_ref(2*i,:)];
end

X = [XYplot_sim(1,:); X];
Y = [XYplot_sim(2,:); Y];   
Vx0 = Velocity_sim*cos(Heading_sim);
Vy0 = Velocity_sim*sin(Heading_sim);
Yaw0 = Heading_sim;

[Velocity_updated, Heading_updated] = P2YV(0,0, T , X , Y , Vx0 , Vy0 , Yaw0, Np, 0, 0 );
end

== matlab function ISReferenceApplication/Subsystem_2/gate2 ==
  data: select_MPC input; state_MPC output; select_overlap input; state_overlap output; select_overlap2 input
function [state_MPC, state_overlap] = gate(select_MPC, select_overlap, select_overlap2)
model_num = 2;
if select_MPC == model_num
    state_MPC = 1;
else
    state_MPC = 0;
end
if select_overlap == model_num || select_overlap2 == model_num
    state_overlap = 1;
else
    state_overlap = 0;
end
end

== matlab function ISReferenceApplication/Subsystem_3/Subsystem/YV_update/YV_update ==
  data: XYplot_ref input; Velocity_updated output; XYplot_sim input; Velocity_sim input; Heading_sim input; Ts input; Tsim input; Heading_updated output
function [Velocity_updated, Heading_updated] = VY_update(XYplot_ref, XYplot_sim, Velocity_sim, Heading_sim, Ts, Tsim)
Np = 6;
 disp(sprintf('Simulation time : %2.1f sec',Tsim)) 
 Heading_updated = zeros(Np,1); Velocity_updated = zeros(Np,1);
coder.extrinsic('P2YV');
T = []; 
for j = 1:Np+1
    T = [T; Tsim+(j-1)*Ts];
end
X = [];
for i = 1:Np
    X = [X; XYplot_ref(2*i-1,:)];
end
Y = [];
for i = 1:Np
    Y = [Y; XYplot_ref(2*i,:)];
end

X = [XYplot_sim(1,:); X];
Y = [XYplot_sim(2,:); Y];   
Vx0 = Velocity_sim*cos(Heading_sim);
Vy0 = Velocity_sim*sin(Heading_sim);
Yaw0 = Heading_sim;

[Velocity_updated, Heading_updated] = P2YV(0,0, T , X , Y , Vx0 , Vy0 , Yaw0, Np, 0, 0 );
end

== matlab function ISReferenceApplication/Subsystem_3/gate3 ==
  data: select_MPC input; state_MPC output; select_overlap input; state_overlap output; select_overlap2 input
function [state_MPC, state_overlap] = gate(select_MPC, select_overlap, select_overlap2)
model_num = 3;
if select_MPC == model_num
    state_MPC = 1;
else
    state_MPC = 0;
end
if select_overlap == model_num || select_overlap2 == model_num
    state_overlap = 1;
else
    state_overlap = 0;
end
end

== matlab function ISReferenceApplication/Subsystem_4/Subsystem/VH2P/YV2P ==
  data: Velocity input; LastVelocity input; Yaw input; LastYaw input; Tsim input; LastTsim input; Lastpostion input; Position output
function Position  = YV2P(Velocity, LastVelocity, Yaw, LastYaw, Tsim, LastTsim, Lastpostion)
if Tsim >= 0.1
    Position = zeros(2,1);
    X0 = Lastpostion(1,:); Y0 = Lastpostion(2,:);
    Vx = [LastVelocity*cos(LastYaw); Velocity*cos(Yaw)];
    Vy = [LastVelocity*sin(LastYaw); Velocity*sin(Yaw)];
    Yaw_sim = [LastYaw; Yaw];
    T_sample =[LastTsim; Tsim];
    [ X_tmp, Y_tmp] = YV2P( T_sample, X0, Y0, Vx, Vy, Yaw_sim, zeros(2,1) );
    Position = [X_tmp(end,:); Y_tmp(end,:)];
else
    Position = [0; 0];
end

end

== matlab function ISReferenceApplication/Subsystem_4/Subsystem/YV_update/YV_update ==
  data: XYplot_ref input; Velocity_updated output; XYplot_sim input; Velocity_sim input; Heading_sim input; Ts input; Tsim input; Heading_updated output
function [Velocity_updated, Heading_updated] = VY_update(XYplot_ref, XYplot_sim, Velocity_sim, Heading_sim, Ts, Tsim)
Np = 6;
 disp(sprintf('Simulation time : %2.1f sec',Tsim)) 
 Heading_updated = zeros(Np,1); Velocity_updated = zeros(Np,1);
coder.extrinsic('P2YV');
T = []; 
for j = 1:Np+1
    T = [T; Tsim+(j-1)*Ts];
end
X = [];
for i = 1:Np
    X = [X; XYplot_ref(2*i-1,:)];
end
Y = [];
for i = 1:Np
    Y = [Y; XYplot_ref(2*i,:)];
end

X = [XYplot_sim(1,:); X];
Y = [XYplot_sim(2,:); Y];   
Vx0 = Velocity_sim*cos(Heading_sim);
Vy0 = Velocity_sim*sin(Heading_sim);
Yaw0 = Heading_sim;

[Velocity_updated, Heading_updated] = P2YV(0,0, T , X , Y , Vx0 , Vy0 , Yaw0, Np, 0, 0 );
end

== matlab function ISReferenceApplication/Subsystem_4/gate4 ==
  data: select_MPC input; state_MPC output; select_overlap input; state_overlap output; select_overlap2 input
function [state_MPC, state_overlap] = gate(select_MPC, select_overlap, select_overlap2)
model_num = 4;
if select_MPC == model_num
    state_MPC = 1;
else
    state_MPC = 0;
end
if select_overlap == model_num || select_overlap2 == model_num
    state_overlap = 1;
else
    state_overlap = 0;
end
end

== matlab function ISReferenceApplication/Subsystem_5/Subsystem/VH2P/YV2P ==
  data: Velocity input; LastVelocity input; Yaw input; LastYaw input; Tsim input; LastTsim input; Lastpostion input; Position output
function Position  = YV2P(Velocity, LastVelocity, Yaw, LastYaw, Tsim, LastTsim, Lastpostion)
if Tsim >= 0.1
    Position = zeros(2,1);
    X0 = Lastpostion(1,:); Y0 = Lastpostion(2,:);
    Vx = [LastVelocity*cos(LastYaw); Velocity*cos(Yaw)];
    Vy = [LastVelocity*sin(LastYaw); Velocity*sin(Yaw)];
    Yaw_sim = [LastYaw; Yaw];
    T_sample =[LastTsim; Tsim];
    [ X_tmp, Y_tmp] = YV2P( T_sample, X0, Y0, Vx, Vy, Yaw_sim, zeros(2,1) );
    Position = [X_tmp(end,:); Y_tmp(end,:)];
else
    Position = [0; 0];
end

end

== matlab function ISReferenceApplication/Subsystem_5/Subsystem/YV_update/YV_update ==
  data: XYplot_ref input; Velocity_updated output; XYplot_sim input; Velocity_sim input; Heading_sim input; Ts input; Tsim input; Heading_updated output
function [Velocity_updated, Heading_updated] = VY_update(XYplot_ref, XYplot_sim, Velocity_sim, Heading_sim, Ts, Tsim)
Np = 6;
 disp(sprintf('Simulation time : %2.1f sec',Tsim)) 
 Heading_updated = zeros(Np,1); Velocity_updated = zeros(Np,1);
coder.extrinsic('P2YV');
T = []; 
for j = 1:Np+1
    T = [T; Tsim+(j-1)*Ts];
end
X = [];
for i = 1:Np
    X = [X; XYplot_ref(2*i-1,:)];
end
Y = [];
for i = 1:Np
    Y = [Y; XYplot_ref(2*i,:)];
end

X = [XYplot_sim(1,:); X];
Y = [XYplot_sim(2,:); Y];   
Vx0 = Velocity_sim*cos(Heading_sim);
Vy0 = Velocity_sim*sin(Heading_sim);
Yaw0 = Heading_sim;

[Velocity_updated, Heading_updated] = P2YV(0,0, T , X , Y , Vx0 , Vy0 , Yaw0, Np, 0, 0 );
end

== matlab function ISReferenceApplication/Subsystem_5/gate5 ==
  data: select_MPC input; state_MPC output; select_overlap input; state_overlap output; select_overlap2 input
function [state_MPC, state_overlap] = gate(select_MPC, select_overlap, select_overlap2)
model_num = 5;
if select_MPC == model_num
    state_MPC = 1;
else
    state_MPC = 0;
end
if select_overlap == model_num || select_overlap2 == model_num
    state_overlap = 1;
else
    state_overlap = 0;
end
end

== matlab function ISReferenceApplication/VH2P/YV2P ==
  data: Velocity input; LastVelocity input; Yaw input; LastYaw input; Tsim input; LastTsim input; Lastpostion input; Position output
function Position  = YV2P(Velocity, LastVelocity, Yaw, LastYaw, Tsim, LastTsim, Lastpostion)
if Tsim >= 0.1
    Position = zeros(2,1);
    X0 = Lastpostion(1,:); Y0 = Lastpostion(2,:);
    Vx = [LastVelocity*cos(LastYaw); Velocity*cos(Yaw)];
    Vy = [LastVelocity*sin(LastYaw); Velocity*sin(Yaw)];
    Yaw_sim = [LastYaw; Yaw];
    T_sample =[LastTsim; Tsim];
    [ X_tmp, Y_tmp] = YV2P( T_sample, X0, Y0, Vx, Vy, Yaw_sim, zeros(2,1) );
    Position = [X_tmp(end,:); Y_tmp(end,:)];
else
    Position = [0; 0];
end

end

== matlab function ISReferenceApplication/Subsystem_6/gate6 ==
  data: select_MPC input; state_MPC output; select_overlap input; state_overlap output; select_overlap2 input
function [state_MPC, state_overlap] = gate(select_MPC, select_overlap, select_overlap2)
model_num = 6;
if select_MPC == model_num
    state_MPC = 1;
else
    state_MPC = 0;
end
if select_overlap == model_num || select_overlap2 == model_num
    state_overlap = 1;
else
    state_overlap = 0;
end
end

== matlab function ISReferenceApplication/Subsystem_7/Subsystem/VH2P/YV2P ==
  data: Velocity input; LastVelocity input; Yaw input; LastYaw input; Tsim input; LastTsim input; Lastpostion input; Position output
function Position  = YV2P(Velocity, LastVelocity, Yaw, LastYaw, Tsim, LastTsim, Lastpostion)
if Tsim >= 0.1
    Position = zeros(2,1);
    X0 = Lastpostion(1,:); Y0 = Lastpostion(2,:);
    Vx = [LastVelocity*cos(LastYaw); Velocity*cos(Yaw)];
    Vy = [LastVelocity*sin(LastYaw); Velocity*sin(Yaw)];
    Yaw_sim = [LastYaw; Yaw];
    T_sample =[LastTsim; Tsim];
    [ X_tmp, Y_tmp] = YV2P( T_sample, X0, Y0, Vx, Vy, Yaw_sim, zeros(2,1) );
    Position = [X_tmp(end,:); Y_tmp(end,:)];
else
    Position = [0; 0];
end

end

== matlab function ISReferenceApplication/Subsystem_7/Subsystem/YV_update/YV_update ==
  data: XYplot_ref input; Velocity_updated output; XYplot_sim input; Velocity_sim input; Heading_sim input; Ts input; Tsim input; Heading_updated output
function [Velocity_updated, Heading_updated] = VY_update(XYplot_ref, XYplot_sim, Velocity_sim, Heading_sim, Ts, Tsim)
Np = 6;
 disp(sprintf('Simulation time : %2.1f sec',Tsim)) 
 Heading_updated = zeros(Np,1); Velocity_updated = zeros(Np,1);
coder.extrinsic('P2YV');
T = []; 
for j = 1:Np+1
    T = [T; Tsim+(j-1)*Ts];
end
X = [];
for i = 1:Np
    X = [X; XYplot_ref(2*i-1,:)];
end
Y = [];
for i = 1:Np
    Y = [Y; XYplot_ref(2*i,:)];
end

X = [XYplot_sim(1,:); X];
Y = [XYplot_sim(2,:); Y];   
Vx0 = Velocity_sim*cos(Heading_sim);
Vy0 = Velocity_sim*sin(Heading_sim);
Yaw0 = Heading_sim;

[Velocity_updated, Heading_updated] = P2YV(0,0, T , X , Y , Vx0 , Vy0 , Yaw0, Np, 0, 0 );
end

== matlab function ISReferenceApplication/MATLAB Function2 ==
  data: u input; Ac output; Br output
function [Ac, Br] = choose(u)
Ac = 0; Br = 0;
if u > 0 || u == 0
    Ac = u;
else
    Br = abs(u);
end
end

== matlab function ISReferenceApplication/Subsystem_7/gate7 ==
  data: select_MPC input; state_MPC output; select_overlap input; state_overlap output; select_overlap2 input
function [state_MPC, state_overlap] = gate(select_MPC, select_overlap, select_overlap2)
model_num = 7;
if select_MPC == model_num
    state_MPC = 1;
else
    state_MPC = 0;
end
if select_overlap == model_num || select_overlap2 == model_num
    state_overlap = 1;
else
    state_overlap = 0;
end
end

== matlab function ISReferenceApplication/Subsystem_8/Subsystem/VH2P/YV2P ==
  data: Velocity input; LastVelocity input; Yaw input; LastYaw input; Tsim input; LastTsim input; Lastpostion input; Position output
function Position  = YV2P(Velocity, LastVelocity, Yaw, LastYaw, Tsim, LastTsim, Lastpostion)
if Tsim >= 0.1
    Position = zeros(2,1);
    X0 = Lastpostion(1,:); Y0 = Lastpostion(2,:);
    Vx = [LastVelocity*cos(LastYaw); Velocity*cos(Yaw)];
    Vy = [LastVelocity*sin(LastYaw); Velocity*sin(Yaw)];
    Yaw_sim = [LastYaw; Yaw];
    T_sample =[LastTsim; Tsim];
    [ X_tmp, Y_tmp] = YV2P( T_sample, X0, Y0, Vx, Vy, Yaw_sim, zeros(2,1) );
    Position = [X_tmp(end,:); Y_tmp(end,:)];
else
    Position = [0; 0];
end

end

== matlab function ISReferenceApplication/Subsystem_8/Subsystem/YV_update/YV_update ==
  data: XYplot_ref input; Velocity_updated output; XYplot_sim input; Velocity_sim input; Heading_sim input; Ts input; Tsim input; Heading_updated output
function [Velocity_updated, Heading_updated] = VY_update(XYplot_ref, XYplot_sim, Velocity_sim, Heading_sim, Ts, Tsim)
Np = 6;
 disp(sprintf('Simulation time : %2.1f sec',Tsim)) 
 Heading_updated = zeros(Np,1); Velocity_updated = zeros(Np,1);
coder.extrinsic('P2YV');
T = []; 
for j = 1:Np+1
    T = [T; Tsim+(j-1)*Ts];
end
X = [];
for i = 1:Np
    X = [X; XYplot_ref(2*i-1,:)];
end
Y = [];
for i = 1:Np
    Y = [Y; XYplot_ref(2*i,:)];
end

X = [XYplot_sim(1,:); X];
Y = [XYplot_sim(2,:); Y];   
Vx0 = Velocity_sim*cos(Heading_sim);
Vy0 = Velocity_sim*sin(Heading_sim);
Yaw0 = Heading_sim;

[Velocity_updated, Heading_updated] = P2YV(0,0, T , X , Y , Vx0 , Vy0 , Yaw0, Np, 0, 0 );
end

== matlab function ISReferenceApplication/Subsystem_1/gate1 ==
  data: select_MPC input; state_MPC output; select_overlap input; state_overlap output; select_overlap2 input
function [state_MPC, state_overlap] = gate(select_MPC, select_overlap, select_overlap2)
model_num = 1;
if select_MPC == model_num
    state_MPC = 1;
else
    state_MPC = 0;
end
if select_overlap == model_num || select_overlap2 == model_num
    state_overlap = 1;
else
    state_overlap = 0;
end
end

== matlab function ISReferenceApplication/Subsystem_8/gate8 ==
  data: select_MPC input; state_MPC output; select_overlap input; state_overlap output; select_overlap2 input
function [state_MPC, state_overlap] = gate(select_MPC, select_overlap, select_overlap2)
model_num = 8;
if select_MPC == model_num
    state_MPC = 1;
else
    state_MPC = 0;
end
if select_overlap == model_num || select_overlap2 == model_num
    state_overlap = 1;
else
    state_overlap = 0;
end
end

== matlab function ISReferenceApplication/Subsystem_9/Subsystem/VH2P/YV2P ==
  data: Velocity input; LastVelocity input; Yaw input; LastYaw input; Tsim input; LastTsim input; Lastpostion input; Position output
function Position  = YV2P(Velocity, LastVelocity, Yaw, LastYaw, Tsim, LastTsim, Lastpostion)
if Tsim >= 0.1
    Position = zeros(2,1);
    X0 = Lastpostion(1,:); Y0 = Lastpostion(2,:);
    Vx = [LastVelocity*cos(LastYaw); Velocity*cos(Yaw)];
    Vy = [LastVelocity*sin(LastYaw); Velocity*sin(Yaw)];
    Yaw_sim = [LastYaw; Yaw];
    T_sample =[LastTsim; Tsim];
    [ X_tmp, Y_tmp] = YV2P( T_sample, X0, Y0, Vx, Vy, Yaw_sim, zeros(2,1) );
    Position = [X_tmp(end,:); Y_tmp(end,:)];
else
    Position = [0; 0];
end

end

== matlab function ISReferenceApplication/Subsystem_9/Subsystem/YV_update/YV_update ==
  data: XYplot_ref input; Velocity_updated output; XYplot_sim input; Velocity_sim input; Heading_sim input; Ts input; Tsim input; Heading_updated output
function [Velocity_updated, Heading_updated] = VY_update(XYplot_ref, XYplot_sim, Velocity_sim, Heading_sim, Ts, Tsim)
Np = 6;
 disp(sprintf('Simulation time : %2.1f sec',Tsim)) 
 Heading_updated = zeros(Np,1); Velocity_updated = zeros(Np,1);
coder.extrinsic('P2YV');
T = []; 
for j = 1:Np+1
    T = [T; Tsim+(j-1)*Ts];
end
X = [];
for i = 1:Np
    X = [X; XYplot_ref(2*i-1,:)];
end
Y = [];
for i = 1:Np
    Y = [Y; XYplot_ref(2*i,:)];
end

X = [XYplot_sim(1,:); X];
Y = [XYplot_sim(2,:); Y];   
Vx0 = Velocity_sim*cos(Heading_sim);
Vy0 = Velocity_sim*sin(Heading_sim);
Yaw0 = Heading_sim;

[Velocity_updated, Heading_updated] = P2YV(0,0, T , X , Y , Vx0 , Vy0 , Yaw0, Np, 0, 0 );
end

== matlab function ISReferenceApplication/Subsystem_9/gate9 ==
  data: select_MPC input; state_MPC output; select_overlap input; state_overlap output; select_overlap2 input
function [state_MPC, state_overlap] = gate(select_MPC, select_overlap, select_overlap2)
model_num = 9;
if select_MPC == model_num
    state_MPC = 1;
else
    state_MPC = 0;
end
if select_overlap == model_num || select_overlap2 == model_num
    state_overlap = 1;
else
    state_overlap = 0;
end
end
